simulink model "sis2"  (Simulink 8.0)
settings: Solver=ode45  StartTime=0.0  StopTime=10  RelTol=1e-3
settings Model: Creator=Alunos  LastModifiedBy=Katarina
settings DataIOCC: SignalLoggingSaveFormat=ModelDataLogs
settings DebuggingCC: MultiTaskDSMMsg=warning  MultiTaskCondExecSysMsg=none  StrictBusMsg=None
settings RTWCC: IncludeERTFirstTime=on
settings CodeAppCC: CustomSymbolStrType=$N$R$M_T  InternalIdentifier=Shortened

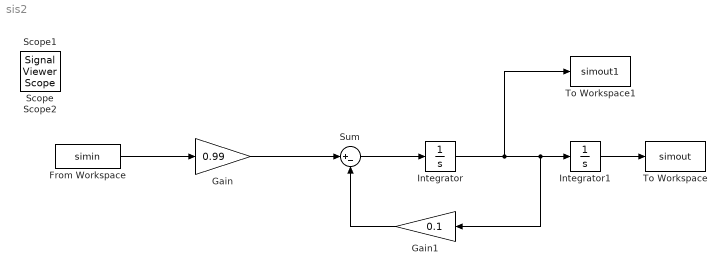
== system sis2 ==
  From Workspace : FromWorkspace  VariableName=simin  SampleTime=0  OutputAfterFinalValue=Setting to zero
  Gain : Gain  Gain=0.99
  Gain1 : Gain  Gain=0.1
  Integrator : Integrator
  Integrator1 : Integrator  InitialCondition=1
  Sum : Sum  Inputs=|+-
  To Workspace : ToWorkspace  VariableName=simout  SampleTime=-1
  To Workspace1 : ToWorkspace  VariableName=simout1  SampleTime=-1
  Scope : SignalViewerScope  IOType=viewer  RefreshTime=0.035000
  Scope1 : SignalViewerScope  IOType=viewer  RefreshTime=0.035000
  Scope2 : SignalViewerScope  IOType=viewer  RefreshTime=0.035000
      settings: SaveName=ScopeData2
  wires:
  Integrator/1 -> To Workspace1/1, Gain1/1, Integrator1/1
  Integrator1/1 -> To Workspace/1
  Sum/1 -> Integrator/1
  From Workspace/1 -> Gain/1
  Gain/1 -> Sum/1
  Gain1/1 -> Sum/2
